simulink model "droop_model_with_current_limitation"  (R2018a)
settings: Solver=ode23tb  StartTime=0.0  StopTime=Tend  RelTol=1e-3
values from neighbouring files (symbols this model uses):
  C_4 = 0.1670*C_b    (= 1.00487241952e-06)    [VSM.m]    (also in dVOC.m; droop.m; droop_with_current_limitation.m; matching.m)
  C_6 = 0.2835*C_b    (= 1.70587623314e-06)    [VSM.m]    (also in dVOC.m; droop.m; droop_with_current_limitation.m; matching.m)
  C_8 = 0.2275*C_b    (= 1.36891302659e-06)    [VSM.m]    (also in dVOC.m; droop.m; droop_with_current_limitation.m; matching.m)
  C_dc = 0.008*(n)    (= 1.6)    [VSM.m]    (also in dVOC.m; droop.m; droop_with_current_limitation.m; matching.m)
  C_f = n*300*10^-6    (= 0.06)    [VSM.m]    (also in dVOC.m; droop.m; droop_with_current_limitation.m; matching.m)
  droop_percentage = 1    [VSM.m]    (also in dVOC.m; droop.m; droop_with_current_limitation.m; matching.m)
  I_b_LV = S_b/(sqrt(3)*V1_rms)    [VSM.m]    (also in dVOC.m; droop.m; droop_with_current_limitation.m = sqrt(2)*S_b/(sqrt(3)*V1_rms); matching.m)
  i_ll = -1.15*(S_b/Vdc_n)-i_loss_dc    [VSM.m]    (also in dVOC.m; droop.m; droop_with_current_limitation.m; matching.m)
  i_ul = 1.15*(S_b/Vdc_n)+i_loss_dc    [VSM.m]    (also in dVOC.m; droop.m; droop_with_current_limitation.m; matching.m)
  idppu = 0.9    [droop_with_current_limitation.m]
  isatpu = 1.2    [droop_with_current_limitation.m]
  k_dc = eta_1/(Vdc_n*m_p)    [VSM.m]    (also in dVOC.m; droop.m; droop_with_current_limitation.m; matching.m)
  K_dP = 2.3*S_b    (= 230000000)    [droop_with_current_limitation.m]
  K_p = (1/Vdc_n)    [VSM.m]    (also in dVOC.m; droop.m; droop_with_current_limitation.m; matching.m)
  K_r = 1/R_dc    [VSM.m]    (also in dVOC.m; droop.m; droop_with_current_limitation.m; matching.m)
  Kff_i = 1    [VSM.m]    (also in dVOC.m; droop.m; droop_with_current_limitation.m; matching.m)
  Kff_v = 1    [VSM.m]    (also in dVOC.m; droop.m; droop_with_current_limitation.m; matching.m)
  Ki_i = (1/n)*1.19    (= 0.00595)    [VSM.m]    (also in dVOC.m; droop.m; droop_with_current_limitation.m; matching.m)
  Ki_v = (n)*1.161022    (= 232.2044)    [VSM.m]    (also in dVOC.m; droop.m; droop_with_current_limitation.m; matching.m)
  ki_v_ac = 4*5.2500e-04    (= 0.0021)    [VSM.m]    (also in dVOC.m = 0.5; droop.m = 0.5; droop_with_current_limitation.m = 0.5; matching.m = 0.5)
  Kp_i = 0.738891    [VSM.m]    (also in dVOC.m; droop.m; droop_with_current_limitation.m; matching.m)
  Kp_v = 0.52    [VSM.m]    (also in dVOC.m; droop.m; droop_with_current_limitation.m; matching.m)
  kp_v_ac = 0.001    [VSM.m]    (also in dVOC.m; droop.m; droop_with_current_limitation.m; matching.m)
  L1_pu = 1*0.0186/m    (= 0.000186)    [VSM.m]    (also in dVOC.m; droop.m; droop_with_current_limitation.m; matching.m)
  L_45 = L_lines(2)    [VSM.m]    (also in dVOC.m; droop.m; droop_with_current_limitation.m; matching.m)
  L_56 = L_lines(3)    [VSM.m]    (also in dVOC.m; droop.m; droop_with_current_limitation.m; matching.m)
  L_67 = L_lines(5)    [VSM.m]    (also in dVOC.m; droop.m; droop_with_current_limitation.m; matching.m)
  L_78 = L_lines(6)    [VSM.m]    (also in dVOC.m; droop.m; droop_with_current_limitation.m; matching.m)
  L_89 = L_lines(8)    [VSM.m]    (also in dVOC.m; droop.m; droop_with_current_limitation.m; matching.m)
  L_94 = L_lines(9)    [VSM.m]    (also in dVOC.m; droop.m; droop_with_current_limitation.m; matching.m)
  L_f = (1/n)*200*10^-6    (= 1e-06)    [VSM.m]    (also in dVOC.m; droop.m; droop_with_current_limitation.m; matching.m)
  m_p = (2*pi*0.5)/(S_b)    (= 3.14159265359e-08)    [VSM.m]    (also in dVOC.m; droop.m; droop_with_current_limitation.m; matching.m)
  n = 200    [VSM.m]    (also in dVOC.m; droop.m; droop_with_current_limitation.m; matching.m)
  ps = base/3    (= 0.75)    [VSM.m]    (also in dVOC.m; droop.m; droop_with_current_limitation.m; matching.m)
  R1_pu = 1*0.00734/m    (= 7.34e-05)    [VSM.m]    (also in dVOC.m; droop.m; droop_with_current_limitation.m; matching.m)
  R_45 = R_lines(2)    [VSM.m]    (also in dVOC.m; droop.m; droop_with_current_limitation.m; matching.m)
  R_56 = R_lines(3)    [VSM.m]    (also in dVOC.m; droop.m; droop_with_current_limitation.m; matching.m)
  R_67 = R_lines(5)    [VSM.m]    (also in dVOC.m; droop.m; droop_with_current_limitation.m; matching.m)
  R_78 = R_lines(6)    [VSM.m]    (also in dVOC.m; droop.m; droop_with_current_limitation.m; matching.m)
  R_89 = R_lines(8)    [VSM.m]    (also in dVOC.m; droop.m; droop_with_current_limitation.m; matching.m)
  R_94 = R_lines(9)    [VSM.m]    (also in dVOC.m; droop.m; droop_with_current_limitation.m; matching.m)
  R_dc = (Vdc_n/(0.05*(S_b)/Vdc_n))    [VSM.m]    (also in dVOC.m; droop.m; droop_with_current_limitation.m; matching.m)
  R_f = 0.001/n    (= 5e-06)    [VSM.m]    (also in dVOC.m; droop.m; droop_with_current_limitation.m; matching.m)
  S_b = 100*(10^6)    (= 100000000)    [VSM.m]    (also in dVOC.m; droop.m; droop_with_current_limitation.m; matching.m)
  S_bt = S_b    (= 100000000)    [VSM.m]    (also in dVOC.m; droop.m; droop_with_current_limitation.m; matching.m)
  T_en = T_load-0.5    (= 24.5)    [VSM.m]    (also in dVOC.m; droop.m; droop_with_current_limitation.m; matching.m)
  T_load = 25    [VSM.m]    (also in dVOC.m; droop.m; droop_with_current_limitation.m; matching.m)
  T_loss = Tend    (= 50)    [dVOC.m]    (also in droop.m; droop_with_current_limitation.m)
  T_ms = 0.001    [dVOC.m]    (also in droop.m; droop_with_current_limitation.m)
  T_s = 1e-4    (= 0.0001)    [VSM.m]    (also in dVOC.m; droop.m; droop_with_current_limitation.m; matching.m)
  tau_dc = 0.05    [VSM.m]    (also in dVOC.m; droop.m; droop_with_current_limitation.m; matching.m)
  tau_g = 5    [VSM.m]    (also in dVOC.m; droop.m; droop_with_current_limitation.m; matching.m)
  V1_rms = 1000    [VSM.m]    (also in dVOC.m; droop.m; droop_with_current_limitation.m; matching.m)
  V2_rms = 13800    [VSM.m]    (also in dVOC.m; droop.m; droop_with_current_limitation.m; matching.m)
  V_m = sqrt(2/3)*V1_rms    [VSM.m]    (also in dVOC.m; droop.m; droop_with_current_limitation.m; matching.m)
  Vdc_n = 3*V_m    [VSM.m]    (also in dVOC.m; droop.m; droop_with_current_limitation.m; matching.m)
  w_b = 2*pi*f_b    (= 314.159265359)    [VSM.m]    (also in dVOC.m; droop.m; droop_with_current_limitation.m; matching.m)
  w_f = 2*pi*5    (= 31.4159265359)    [VSM.m]    (also in dVOC.m; droop.m; droop_with_current_limitation.m; matching.m)
undefined symbols (not defined in the file or in its folder): D1, Delta, i_dc
libraries: powerlib x88, powerlib_meascontrol x22, cstblocks x3, simulink x2, sps_avr x1
(part 1 of 2)
settings Model: SimulationMode=accelerator  ExtModeTrigDuration=100  Creator=TayyebiA  LastModifiedBy=TayyebiA
settings DataIOCC: SaveOutput=off  StateSaveName=tmp_raccel_xout  SignalLoggingName=tmp_raccel_logsout
settings OptimizationCC: EfficientMapNaN2IntZero=off
settings HardwareCC: TargetBitPerPointer=64  TargetBitPerSizeT=64  TargetBitPerPtrDiffT=64  TargetLongLongMode=on  TargetIntDivRoundTo=Zero  TargetEndianess=LittleEndian  TargetWordSize=64  TargetHWDeviceType=MATLAB Host  ProdEqTarget=off
settings CodeAppCC: MaxIdLength=128
settings GRTTargetCC: TargetLangStandard=C89/C90 (ANSI)  CombineOutputUpdateFcns=off  GRTInterface=on

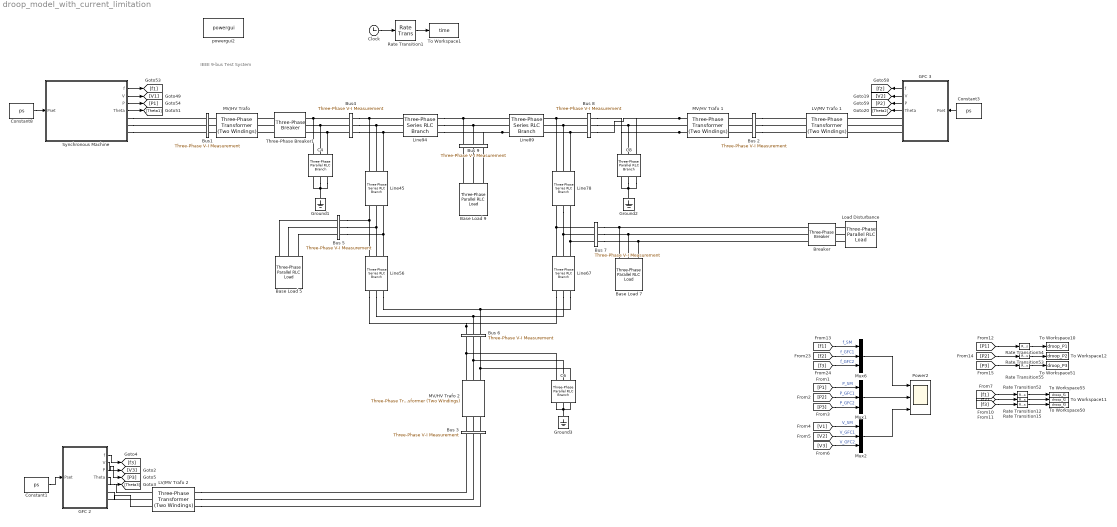
== system droop_model_with_current_limitation ==
  note: IEEE 9-bus Test System
  Base Load 5 : powerlib/Elements/Three-Phase Parallel RLC Load  LConnTagsString=A|B|C  Configuration=Y (grounded)  NominalVoltage=230e3  Vabc=[1e3 1e3 1e3]  Vabcp=[1e3 1e3 1e3]  NominalFrequency=50  UnbalancedPower=off  ActivePower=pl  InductivePower=0  CapacitivePower=0  Pabc=[10e3 9e3 11e3]  QLabc=[100 90 110]  QCabc=[100 90 110]  Pabcp=[10e3 9e3 11e3]  QLabcp=[100 90 110]  QCabcp=[100 90 110]  Measurements=None  LoadType=constant Z
  Base Load 7 : powerlib/Elements/Three-Phase Parallel RLC Load  LConnTagsString=A|B|C  Configuration=Y (grounded)  NominalVoltage=230e3  Vabc=[1e3 1e3 1e3]  Vabcp=[1e3 1e3 1e3]  NominalFrequency=50  UnbalancedPower=off  ActivePower=pl  InductivePower=0  CapacitivePower=0  Pabc=[10e3 9e3 11e3]  QLabc=[100 90 110]  QCabc=[100 90 110]  Pabcp=[10e3 9e3 11e3]  QLabcp=[100 90 110]  QCabcp=[100 90 110]  Measurements=None  LoadType=constant Z
  "Base Load 9 " : powerlib/Elements/Three-Phase Parallel RLC Load  LConnTagsString=A|B|C  Configuration=Y (grounded)  NominalVoltage=230e3  Vabc=[1e3 1e3 1e3]  Vabcp=[1e3 1e3 1e3]  NominalFrequency=50  UnbalancedPower=off  ActivePower=pl  InductivePower=0  CapacitivePower=0  Pabc=[10e3 9e3 11e3]  QLabc=[100 90 110]  QCabc=[100 90 110]  Pabcp=[10e3 9e3 11e3]  QLabcp=[100 90 110]  QCabcp=[100 90 110]  Measurements=None  LoadType=constant Z
  Breaker : powerlib/Elements/Three-Phase Breaker  InitialState=open  SwitchA=on  SwitchB=on  SwitchC=on  SwitchTimes=[T_load]  External=off  BreakerResistance=0.01  SnubberResistance=1e6  SnubberCapacitance=inf  Measurements=None
  Bus 2 : powerlib/Measurements/Three-Phase V-I Measurement  VoltageMeasurement=no  SetLabelV=on  LabelV=Vabc_8  Vpu=on  VpuLL=off  CurrentMeasurement=no  SetLabelI=on  LabelI=Iabc_8  Ipu=on  Pbase=S_b  Vbase=V_b  OutputType=Complex  PhasorSimulation=off  PSBequivalent=0
  Bus 3 : powerlib/Measurements/Three-Phase V-I Measurement  VoltageMeasurement=no  SetLabelV=off  LabelV=Vabc_6  Vpu=off  VpuLL=off  CurrentMeasurement=no  SetLabelI=off  LabelI=Iabc_6  Ipu=off  Pbase=S_b  Vbase=V_b  OutputType=Complex  PhasorSimulation=off  PSBequivalent=0
  Bus 5 : powerlib/Measurements/Three-Phase V-I Measurement  VoltageMeasurement=no  SetLabelV=on  LabelV=Vabc_5  Vpu=on  VpuLL=off  CurrentMeasurement=no  SetLabelI=on  LabelI=Iabc_5  Ipu=on  Pbase=S_b  Vbase=V_b  OutputType=Complex  PhasorSimulation=off  PSBequivalent=0
  Bus 6 : powerlib/Measurements/Three-Phase V-I Measurement  VoltageMeasurement=no  SetLabelV=off  LabelV=Vabc_6  Vpu=off  VpuLL=off  CurrentMeasurement=no  SetLabelI=off  LabelI=Iabc_6  Ipu=off  Pbase=S_b  Vbase=V_b  OutputType=Complex  PhasorSimulation=off  PSBequivalent=0
  Bus 7 : powerlib/Measurements/Three-Phase V-I Measurement  VoltageMeasurement=no  SetLabelV=on  LabelV=Vabc_5  Vpu=on  VpuLL=off  CurrentMeasurement=no  SetLabelI=on  LabelI=Iabc_5  Ipu=on  Pbase=S_b  Vbase=V_b  OutputType=Complex  PhasorSimulation=off  PSBequivalent=0
  Bus 8 : powerlib/Measurements/Three-Phase V-I Measurement  VoltageMeasurement=no  SetLabelV=on  LabelV=Vabc_8  Vpu=on  VpuLL=off  CurrentMeasurement=no  SetLabelI=on  LabelI=Iabc_8  Ipu=on  Pbase=S_b  Vbase=V_b  OutputType=Complex  PhasorSimulation=off  PSBequivalent=0
  Bus 9 : powerlib/Measurements/Three-Phase V-I Measurement  VoltageMeasurement=no  SetLabelV=on  LabelV=Vabc_9  Vpu=on  VpuLL=off  CurrentMeasurement=no  SetLabelI=on  LabelI=Iabc_9  Ipu=on  Pbase=S_b  Vbase=V_b  OutputType=Complex  PhasorSimulation=off  PSBequivalent=0
  Bus1 : powerlib/Measurements/Three-Phase V-I Measurement  VoltageMeasurement=no  SetLabelV=on  LabelV=Vabc_1  Vpu=on  VpuLL=off  CurrentMeasurement=no  SetLabelI=on  LabelI=Iabc_1  Ipu=on  Pbase=S_b  Vbase=V_b  OutputType=Complex  PhasorSimulation=off  PSBequivalent=0
  Bus4 : powerlib/Measurements/Three-Phase V-I Measurement  VoltageMeasurement=no  SetLabelV=on  LabelV=Vabc_4  Vpu=on  VpuLL=off  CurrentMeasurement=no  SetLabelI=on  LabelI=Iabc_4  Ipu=on  Pbase=S_b  Vbase=V_b  OutputType=Complex  PhasorSimulation=off  PSBequivalent=0
  C4 : powerlib/Elements/Three-Phase Parallel RLC Branch  LConnTagsString=A|B|C  RConnTagsString=A|B|C  BranchType=C  Resistance=1  Inductance=1e-3  Capacitance=C_4  Measurements=None
      settings: SourceProductName=Simscape Power Systems  SourceProductBaseCode=PS
  C6 : powerlib/Elements/Three-Phase Parallel RLC Branch  LConnTagsString=A|B|C  RConnTagsString=A|B|C  BranchType=C  Resistance=1  Inductance=1e-3  Capacitance=C_6  Measurements=None
      settings: SourceProductName=Simscape Power Systems  SourceProductBaseCode=PS
  C8 : powerlib/Elements/Three-Phase Parallel RLC Branch  LConnTagsString=A|B|C  RConnTagsString=A|B|C  BranchType=C  Resistance=1  Inductance=1e-3  Capacitance=C_8  Measurements=None
      settings: SourceProductName=Simscape Power Systems  SourceProductBaseCode=PS
  Clock : Clock
  Constant1 : Constant  Value=ps
  Constant3 : Constant  Value=ps
  Constant8 : Constant  Value=ps
  GFC 2 : Subsystem
  GFC 3 : Subsystem
  Ground1 : powerlib/Elements/Ground  LConnTagsString=a
  Ground2 : powerlib/Elements/Ground  LConnTagsString=a
  Ground3 : powerlib/Elements/Ground  LConnTagsString=a
  LV/MV Trafo 1 : powerlib/Elements/Three-Phase Transformer (Two Windings)  Winding1Connection=Yg  Winding2Connection=Yg  CoreType=Three single-phase transformers  SetSaturation=off  Hysteresis=off  DataFile='hysteresis'  SetInitialFlux=off  Measurements=None  UNITS=pu  NominalPower=[S_bt 50 ]  Winding1="[ V1_rms R1_pu  L1_pu]"  Winding2=[ V2_rms R1_pu L1_pu]  Rm=Rm_pu  Lm=Lm_pu  L0=0.5  Saturation="[ 0,0  ;  0.005,1.2  ;  1.0,1.4 ]"  InitialFluxes=[ 0.8 , -0.8 , 0.7 ]  MoreParameters=off  BreakLoop=off  DataType=off  TransfoNumber=0
  LV/MV Trafo 2 : powerlib/Elements/Three-Phase Transformer (Two Windings)  Winding1Connection=Yg  Winding2Connection=Yg  CoreType=Three single-phase transformers  SetSaturation=off  Hysteresis=off  DataFile='hysteresis'  SetInitialFlux=off  Measurements=None  UNITS=pu  NominalPower=[ S_bt 50 ]  Winding1="[ V1_rms R1_pu  L1_pu]"  Winding2=[ V2_rms R1_pu L1_pu]  Rm=Rm_pu  Lm=Lm_pu  L0=0.5  Saturation="[ 0,0  ;  0.005,1.2  ;  1.0,1.4 ]"  InitialFluxes=[ 0.8 , -0.8 , 0.7 ]  MoreParameters=off  BreakLoop=off  DataType=off  TransfoNumber=0
  Line45 : powerlib/Elements/Three-Phase Series RLC Branch  LConnTagsString=A|B|C  RConnTagsString=A|B|C  BranchType=RL  Resistance=R_45  Inductance=L_45  Capacitance=0  Measurements=None
  Line56 : powerlib/Elements/Three-Phase Series RLC Branch  LConnTagsString=A|B|C  RConnTagsString=A|B|C  BranchType=RL  Resistance=R_56  Inductance=L_56  Capacitance=0  Measurements=None
  Line67 : powerlib/Elements/Three-Phase Series RLC Branch  LConnTagsString=A|B|C  RConnTagsString=A|B|C  BranchType=RL  Resistance=R_67  Inductance=L_67  Capacitance=0  Measurements=None
  Line78 : powerlib/Elements/Three-Phase Series RLC Branch  LConnTagsString=A|B|C  RConnTagsString=A|B|C  BranchType=RL  Resistance=R_78  Inductance=L_78  Capacitance=0  Measurements=None
  Line89 : powerlib/Elements/Three-Phase Series RLC Branch  LConnTagsString=A|B|C  RConnTagsString=A|B|C  BranchType=RL  Resistance=R_89  Inductance=L_89  Capacitance=0  Measurements=None
  Line94 : powerlib/Elements/Three-Phase Series RLC Branch  LConnTagsString=A|B|C  RConnTagsString=A|B|C  BranchType=RL  Resistance=R_94  Inductance=L_94  Capacitance=0  Measurements=None
  Load Disturbance : powerlib/Elements/Three-Phase Parallel RLC Load  LConnTagsString=A|B|C  Configuration=Y (grounded)  NominalVoltage=230e3  Vabc=[1e3 1e3 1e3]  Vabcp=[1e3 1e3 1e3]  NominalFrequency=50  UnbalancedPower=off  ActivePower=load_step  InductivePower=0  CapacitivePower=0  Pabc=[10e3 9e3 11e3]  QLabc=[100 90 110]  QCabc=[100 90 110]  Pabcp=[10e3 9e3 11e3]  QLabcp=[100 90 110]  QCabcp=[100 90 110]  Measurements=None  LoadType=constant Z
  "MV/HV Trafo " : powerlib/Elements/Three-Phase Transformer (Two Windings)  Winding1Connection=Delta (D1)  Winding2Connection=Yg  CoreType=Three single-phase transformers  SetSaturation=off  Hysteresis=off  DataFile='hysteresis'  SetInitialFlux=off  Measurements=None  UNITS=pu  NominalPower=[ 210e6 50 ]  Winding1="[V2_rms 0.0027  0.08]"  Winding2=[230e3 0.0027 0.08]  Rm=500  Lm=500  L0=0.5  Saturation="[ 0,0  ;  0.005,1.2  ;  1.0,1.4 ]"  InitialFluxes=[ 0.8 , -0.8 , 0.7 ]  MoreParameters=off  BreakLoop=off  DataType=off  TransfoNumber=0
  "MV/HV Trafo 1 " : powerlib/Elements/Three-Phase Transformer (Two Windings)  Winding1Connection=Yg  Winding2Connection=Yg  CoreType=Three single-phase transformers  SetSaturation=off  Hysteresis=off  DataFile='hysteresis'  SetInitialFlux=off  Measurements=None  UNITS=pu  NominalPower=[ 210e6 50 ]  Winding1=[V2_rms 0.0027 0.08]  Winding2=[ 230e3 0.0027 0.08]  Rm=500  Lm=500  L0=0.5  Saturation="[ 0,0  ;  0.005,1.2  ;  1.0,1.4 ]"  InitialFluxes=[ 0.8 , -0.8 , 0.7 ]  MoreParameters=off  BreakLoop=off  DataType=off  TransfoNumber=0
  "MV/HV Trafo 2 " : powerlib/Elements/Three-Phase Transformer (Two Windings)  Winding1Connection=Yg  Winding2Connection=Yg  CoreType=Three single-phase transformers  SetSaturation=off  Hysteresis=off  DataFile='hysteresis'  SetInitialFlux=off  Measurements=None  UNITS=pu  NominalPower=[ 210e6 50 ]  Winding1=[V2_rms 0.0027 0.08]  Winding2=[230e3 0.0027 0.08]  Rm=500  Lm=500  L0=0.5  Saturation="[ 0,0  ;  0.005,1.2  ;  1.0,1.4 ]"  InitialFluxes=[ 0.8 , -0.8 , 0.7 ]  MoreParameters=off  BreakLoop=off  DataType=off  TransfoNumber=0
  Mux1 : Mux  Inputs=3
  Mux2 : Mux  Inputs=3
  Mux6 : Mux  Inputs=3
  Power2 : Scope  NumInputPorts=3
  Rate Transition1 : RateTransition  OutPortSampleTime=0.001
  Rate Transition{12,15,52..55} (6 alike) : RateTransition  OutPortSampleTime=T_ms
  Synchronous Machine : Subsystem
  Three-Phase Breaker1 : powerlib/Elements/Three-Phase Breaker  InitialState=closed  SwitchA=on  SwitchB=on  SwitchC=on  SwitchTimes=[T_loss]  External=off  BreakerResistance=1  SnubberResistance=1e6  SnubberCapacitance=inf  Measurements=None
  To Workspace1 : ToWorkspace  VariableName=time  SampleTime=T_ms
  To Workspace10 : ToWorkspace  VariableName=droop_P1  SampleTime=-1
  To Workspace11 : ToWorkspace  VariableName=droop_f2  SampleTime=-1
  To Workspace12 : ToWorkspace  VariableName=droop_P2  SampleTime=-1
  To Workspace50 : ToWorkspace  VariableName=droop_f3  SampleTime=-1
  To Workspace51 : ToWorkspace  VariableName=droop_P3  SampleTime=-1
  To Workspace55 : ToWorkspace  VariableName=droop_f1  SampleTime=-1
  powergui2 : powerlib/powergui  Priority=1  SimulationMode=Discrete  SampleTime=T_s  frequency=50  Iterations=50  frequencyindice=0  Pbase=100e6  ErrMax=0.0001  UnitsV=kV  UnitsW=MW  buscounter=0  FunctionMessages=off  echomessages=off  EnableUseOfTLC=off  CurrentSourceSwitches=off  DisableSnubberDevices=off  DisableRonSwitches=off  DisableVfSwitches=off  DisplayEquations=off  SolverType=Tustin/Backward Euler (TBE)  Interpol=off  ExternalGateDelay=off  methode=off  Ts=100  x0status=blocks  SPID=off  SwTol=0  HookPort=off  RestoreLinks=warning  ResistiveCurrentMeasurement=off  Frange=[0:2:500]  Ylog=off  Xlog=on  ShowGrid=off  save=off  variable=ZData  structure=0  ZoomFFT=off  StartTime=0.0  cycles=1  DisplayStyle=1  fundamental=60  FreqAxis=off  MaxFrequency=1000  frequencyindicesteady=1  RmsSteady=1  display=off
  wires:
  Constant3/1 -> GFC 3/1(Pset)
  Constant8/1 -> Synchronous Machine/1(Pset)
  Synchronous Machine/1(f) -> [f1]
  Synchronous Machine/2(V) -> [V1]
  Synchronous Machine/3(P) -> [P1]
  Synchronous Machine/4(Theta) -> [Theta1]
  [f1] -> Mux6/1  "f_SM"
  [f2] -> Mux6/2  "f_GFC1"
  [f3] -> Mux6/3  "f_GFC2"
  [P1] -> Mux1/1  "P_SM"
  [P3] -> Mux1/3  "P_GFC2"
  [P2] -> Mux1/2  "P_GFC1"
  [V2] -> Mux2/2  "V_GFC1"
  [V1] -> Mux2/1  "V_SM"
  [V3] -> Mux2/3  "V_GFC2"
  Mux6/1 -> Power2/1
  Mux1/1 -> Power2/2
  Mux2/1 -> Power2/3
  GFC 3/1(f) -> [f2]
  GFC 3/2(V) -> [V2]
  GFC 3/3(P) -> [P2]
  GFC 3/4(Theta) -> [Theta2]
  GFC 2/1(f) -> [f3]
  GFC 2/2(V) -> [V3]
  GFC 2/3(P) -> [P3]
  Constant1/1 -> GFC 2/1(Pset)
  GFC 2/4(Theta) -> [Theta3]
  [P3] -> Rate Transition55/1
  Rate Transition54/1 -> To Workspace10/1
  Rate Transition55/1 -> To Workspace51/1
  Rate Transition52/1 -> To Workspace55/1
  Rate Transition15/1 -> To Workspace50/1
  Rate Transition12/1 -> To Workspace11/1
  [f2] -> Rate Transition12/1
  [f3] -> Rate Transition15/1
  Rate Transition53/1 -> To Workspace12/1
  [P1] -> Rate Transition54/1
  [f1] -> Rate Transition52/1
  [P2] -> Rate Transition53/1
  Clock/1 -> Rate Transition1/1
  Rate Transition1/1 -> To Workspace1/1
  connections:
  "MV/HV Trafo 2 "/RConn2 -- Bus 6/RConn2 -- C6/LConn2
  Breaker/LConn2 -- Base Load 7/LConn2 -- Bus 7/LConn2
  Bus 8/RConn2 -- Line78/LConn2 -- Line89/RConn2
  GFC 3/RConn3 -- LV/MV Trafo 1/LConn1
  "MV/HV Trafo 1 "/RConn3 -- C8/LConn3 -- Bus 8/LConn3
  Line94/RConn2 -- Line89/LConn2 -- Bus 9/RConn2
  Bus 6/LConn1 -- Line56/RConn1 -- Line67/RConn1
  Breaker/LConn3 -- Base Load 7/LConn3 -- Bus 7/LConn3
  Line67/LConn1 -- Bus 7/RConn1 -- Line78/RConn1
  Line56/LConn3 -- Bus 5/LConn3 -- Line45/RConn3
  Bus 9/RConn3 -- Line89/LConn1 -- Line94/RConn1
  C4/RConn2 -- C4/RConn1 -- C4/RConn3 -- Ground1/LConn1
  "MV/HV Trafo 1 "/RConn1 -- C8/LConn1 -- Bus 8/LConn1
  Bus 8/LConn2 -- C8/LConn2 -- "MV/HV Trafo 1 "/RConn2
  C8/RConn3 -- Ground2/LConn1 -- C8/RConn1 -- C8/RConn2
  Line67/RConn2 -- Line56/RConn2 -- Bus 6/LConn2
  C4/LConn1 -- Three-Phase Breaker1/RConn1 -- Bus4/RConn1
  Bus4/LConn1 -- Line45/LConn1 -- Line94/LConn1
  C6/LConn3 -- Bus 6/RConn3 -- "MV/HV Trafo 2 "/RConn3
  GFC 3/RConn1 -- LV/MV Trafo 1/LConn3
  "MV/HV Trafo 2 "/RConn1 -- Bus 6/RConn1 -- C6/LConn1
  Bus4/LConn2 -- Line45/LConn2 -- Line94/LConn2
  Bus 8/RConn3 -- Line78/LConn3 -- Line89/RConn3
  Bus 8/RConn1 -- Line78/LConn1 -- Line89/RConn1
  Bus4/RConn3 -- Three-Phase Breaker1/RConn3 -- C4/LConn3
  Line56/LConn1 -- Bus 5/LConn1 -- Line45/RConn1
  Line89/LConn3 -- Bus 9/RConn1 -- Line94/RConn3
  Line67/RConn3 -- Line56/RConn3 -- Bus 6/LConn3
  GFC 3/RConn2 -- LV/MV Trafo 1/LConn2
  Bus4/LConn3 -- Line45/LConn3 -- Line94/LConn3
  Bus4/RConn2 -- Three-Phase Breaker1/RConn2 -- C4/LConn2
  Line56/LConn2 -- Bus 5/LConn2 -- Line45/RConn2
  "Base Load 9 "/LConn1 -- Bus 9/LConn3
  Base Load 5/LConn3 -- Bus 5/RConn3
  "Base Load 9 "/LConn3 -- Bus 9/LConn1
  Base Load 5/LConn1 -- Bus 5/RConn1
  Base Load 5/LConn2 -- Bus 5/RConn2
  "Base Load 9 "/LConn2 -- Bus 9/LConn2
  Load Disturbance/LConn3 -- Breaker/RConn3
  Load Disturbance/LConn2 -- Breaker/RConn2
  Load Disturbance/LConn1 -- Breaker/RConn1
  Bus1/LConn1 -- "MV/HV Trafo "/LConn1
  Bus1/LConn2 -- "MV/HV Trafo "/LConn2
  Bus1/LConn3 -- "MV/HV Trafo "/LConn3
  Synchronous Machine/RConn1 -- Bus1/RConn1
  Synchronous Machine/RConn2 -- Bus1/RConn2
  Synchronous Machine/RConn3 -- Bus1/RConn3
  LV/MV Trafo 2/RConn1 -- Bus 3/RConn1
  LV/MV Trafo 2/RConn2 -- Bus 3/RConn2
  LV/MV Trafo 2/RConn3 -- Bus 3/RConn3
  Bus 3/LConn1 -- "MV/HV Trafo 2 "/LConn1
  Bus 3/LConn2 -- "MV/HV Trafo 2 "/LConn2
  Bus 3/LConn3 -- "MV/HV Trafo 2 "/LConn3
  Bus 2/LConn1 -- LV/MV Trafo 1/RConn3
  Bus 2/LConn2 -- LV/MV Trafo 1/RConn2
  Bus 2/LConn3 -- LV/MV Trafo 1/RConn1
  Bus 2/RConn3 -- "MV/HV Trafo 1 "/LConn1
  Bus 2/RConn2 -- "MV/HV Trafo 1 "/LConn2
  Bus 2/RConn1 -- "MV/HV Trafo 1 "/LConn3
  Breaker/LConn1 -- Bus 7/LConn1 -- Base Load 7/LConn1
  Line67/LConn3 -- Bus 7/RConn3 -- Line78/RConn3
  Line78/RConn2 -- Bus 7/RConn2 -- Line67/LConn2
  C6/RConn1 -- C6/RConn3 -- Ground3/LConn1 -- C6/RConn2
  GFC 2/RConn1 -- LV/MV Trafo 2/LConn1
  GFC 2/RConn2 -- LV/MV Trafo 2/LConn2
  GFC 2/RConn3 -- LV/MV Trafo 2/LConn3
  Three-Phase Breaker1/LConn1 -- "MV/HV Trafo "/RConn1
  Three-Phase Breaker1/LConn2 -- "MV/HV Trafo "/RConn2
  Three-Phase Breaker1/LConn3 -- "MV/HV Trafo "/RConn3

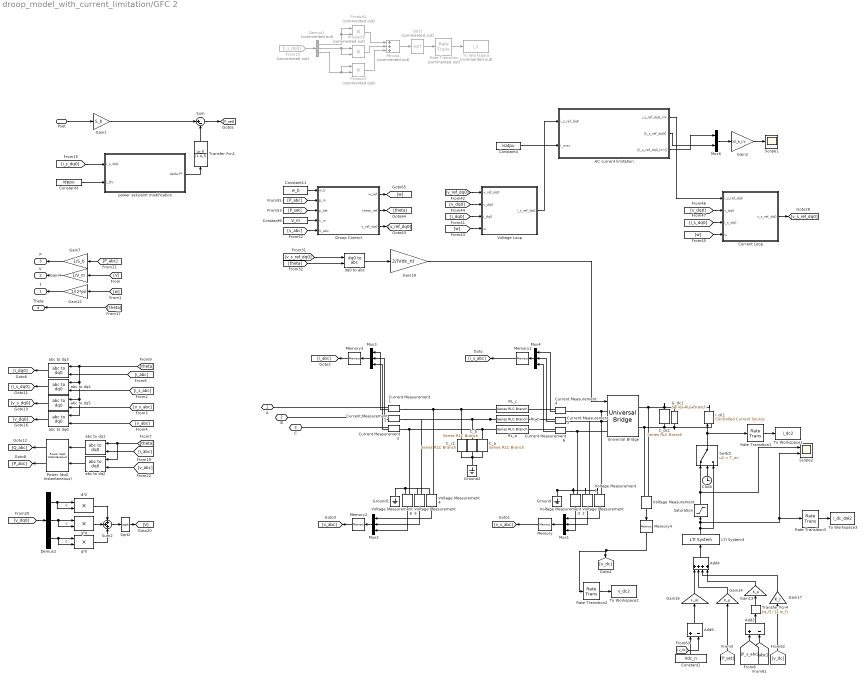
== system droop_model_with_current_limitation/GFC 2 ==
  Pset : Inport
  AC current limitation : Subsystem
  Add2 : Sum  Inputs=+-
  Add4 : Sum  Inputs=++++
  Add6 : Sum  Inputs=+-
  C_a : powerlib/Elements/Series RLC Branch  LConnTagsString=__new0  RConnTagsString=__new0  BranchType=C  Resistance=1  Inductance=1e-3  SetiL0=off  InitialCurrent=0  Capacitance=C_f  Setx0=off  InitialVoltage=165  Measurements=None
  C_b : powerlib/Elements/Series RLC Branch  LConnTagsString=__new0  RConnTagsString=__new0  BranchType=C  Resistance=1  Inductance=1e-3  SetiL0=off  InitialCurrent=0  Capacitance=C_f  Setx0=off  InitialVoltage=165  Measurements=None
  C_c1 : powerlib/Elements/Series RLC Branch  LConnTagsString=__new0  RConnTagsString=__new0  BranchType=C  Resistance=1  Inductance=1e-3  SetiL0=off  InitialCurrent=0  Capacitance=C_f  Setx0=off  InitialVoltage=165  Measurements=None
  C_dc1 : powerlib/Elements/Series RLC Branch  LConnTagsString=__new0  RConnTagsString=__new0  BranchType=C  Resistance=0.01  Inductance=1e-3  SetiL0=off  InitialCurrent=0  Capacitance=C_dc  Setx0=off  InitialVoltage=Vdc_n  Measurements=None
  Clock : Clock
  Constant1 : Constant  Value=Vdc_n
  Constant11 : Constant  Value=w_b
  Constant3 : Constant  Value=idppu
  Constant4 : Constant  Value=isatpu
  Constant9 : Constant  Value=V_m
  Current Loop : Subsystem
  Current Measurement{1..6} (6 alike) : powerlib/Measurements/Current Measurement  PhasorSimulation=off  OutputType=Complex  PSBequivalent=0
  Demux1 : Demux  Commented=on  Outputs=3
  Demux2 : Demux  Outputs=3
  Droop Control : Subsystem
  From10 : From  Commented=on  GotoTag=i_s_dq0
  G_dc1 : powerlib/Elements/Series RLC Branch  LConnTagsString=__new0  RConnTagsString=__new0  BranchType=R  Resistance=R_dc  Inductance=1e-3  SetiL0=off  InitialCurrent=0  Capacitance=1e-6  Setx0=off  InitialVoltage=0  Measurements=None
  Gain1 : Gain  Gain=S_b
  Gain12 : Gain  Gain=1/(2*pi)
  Gain13 : Gain  Gain=K_p
  Gain14 : Gain  Gain=K_p
  Gain16 : Gain  Gain=k_dc
  Gain17 : Gain  Gain=K_r
  Gain19 : Gain  Gain=2/(Vdc_n)
  Gain2 : Gain  Gain=1/I_b_LV
  Gain4 : Gain  Gain=1/V_m
  Gain7 : Gain  Gain=1/S_b
  Ground : powerlib/Elements/Ground  LConnTagsString=a
  Ground1 : powerlib/Elements/Ground  LConnTagsString=a
  Ground2 : powerlib/Elements/Ground  LConnTagsString=a
  LTI System3 : cstblocks/LTI System  sys=tf(1,[tau_dc 1])  IC=[]
  Memory{,1..4} (5 alike) : Memory
  Minus4 : Sum  Commented=on  Inputs=+++
  Mux{1..4} (4 alike) : Mux  Inputs=3
  Mux6 : Mux  Inputs=2
  "Power (dq0, Instantaneous)" : powerlib_meascontrol/Measurements/Power (dq0, Instantaneous)
      settings: SourceProductName=Simscape Power Systems  SourceProductBaseCode=PS
  Product1 : Product  Commented=on  RndMeth=Zero
  Product2 : Product  Commented=on  RndMeth=Zero
  Product7 : Product  Commented=on  RndMeth=Zero
  RL_a : powerlib/Elements/Series RLC Branch  LConnTagsString=__new0  RConnTagsString=__new0  BranchType=RL  Resistance=R_f  Inductance=L_f  SetiL0=off  InitialCurrent=0  Capacitance=1e-6  Setx0=off  InitialVoltage=0  Measurements=Branch voltage and current
  RL_b : powerlib/Elements/Series RLC Branch  LConnTagsString=__new0  RConnTagsString=__new0  BranchType=RL  Resistance=R_f  Inductance=L_f  SetiL0=off  InitialCurrent=0  Capacitance=1e-6  Setx0=off  InitialVoltage=0  Measurements=None
  RL_c : powerlib/Elements/Series RLC Branch  LConnTagsString=__new0  RConnTagsString=__new0  BranchType=RL  Resistance=R_f  Inductance=L_f  SetiL0=off  InitialCurrent=0  Capacitance=1e-6  Setx0=off  InitialVoltage=0  Measurements=None
  Rate Transition : RateTransition  Commented=on  OutPortSampleTime=0.001
  Rate Transition1 : RateTransition  OutPortSampleTime=0.001
  Rate Transition2 : RateTransition  OutPortSampleTime=0.001
  Rate Transition3 : RateTransition  OutPortSampleTime=0.001
  Saturation : Saturate  UpperLimit=i_ul  LowerLimit=i_ll
  Scope1 : Scope
  Scope2 : Scope  NumInputPorts=2
  Sqrt1 : Sqrt  Commented=on  SaturateOnIntegerOverflow=on
  Sqrt2 : Sqrt  SaturateOnIntegerOverflow=on
  Sum : Sum  Inputs=|+-
  Sum2 : Sum  Inputs=+++  SaturateOnIntegerOverflow=on  InputSameDT=on  OutDataTypeStr=Inherit: Same as first input
  Switch : Switch  Criteria=u2 > Threshold  Threshold=T_en
  To Workspace : ToWorkspace  Commented=on  VariableName=i_2  SampleTime=-1
  To Workspace1 : ToWorkspace  VariableName=i_dc2  SampleTime=-1
  To Workspace2 : ToWorkspace  VariableName=v_dc2  SampleTime=-1
  To Workspace3 : ToWorkspace  VariableName=i_dc_del2  SampleTime=-1
  Transfer Fcn1 : TransferFcn  Numerator=[w_f]  Denominator=[1 w_f]
  Transfer Fcn4 : TransferFcn  Numerator=[w_f]  Denominator=[1 w_f]
  Universal Bridge : powerlib/Power Electronics/Universal Bridge  Arms=3  SnubberResistance=1e5  SnubberCapacitance=inf  Device=Average-model based VSC  Ron=1e-3  Lon=0  ForwardVoltages="[  0  0  ]"  ForwardVoltage=0  GTOparameters=[ 10e-6 , 20e-6 ]  IGBTparameters=[ 1e-6 , 2e-6 ]  Measurements=None  Measurements_2=None  converterType=Rectifier
  Voltage Loop : Subsystem
  Voltage Measurement{,1..6} (7 alike) : powerlib/Measurements/Voltage Measurement  PhasorSimulation=off  OutputType=Complex  PSBequivalent=0
  abc to dq{1..6} (6 alike) : powerlib_meascontrol/Transformations/abc to dq0  Alignment=90 degrees behind phase A axis
  dq0 to abc : powerlib_meascontrol/Transformations/dq0 to abc  Alignment=90 degrees behind phase A axis
  d²2 : Product  SaturateOnIntegerOverflow=on  RndMeth=Zero  InputSameDT=on  OutDataTypeStr=Inherit: Same as first input
  i_dc1 : powerlib/Electrical Sources/Controlled Current Source  Initialize=off  Source_Type=DC  Amplitude=i_dc  Phase=0  Frequency=0  Measurements=None
  power set-point modification : Subsystem
  q²4 : Product  SaturateOnIntegerOverflow=on  RndMeth=Zero  InputSameDT=on  OutDataTypeStr=Inherit: Same as first input
  q²5 : Product  SaturateOnIntegerOverflow=on  RndMeth=Zero  InputSameDT=on  OutDataTypeStr=Inherit: Same as first input
  A : PMIOPort  Side=Right
  B : PMIOPort  Port=2  Side=Right
  C : PMIOPort  Port=3  Side=Right
  f : Outport
  V : Outport  Port=2
  P : Outport  Port=3
  Theta : Outport  Port=4
  wires:
  Product2/1 -> Minus4/2
  Sqrt1/1 -> Rate Transition/1
  Rate Transition/1 -> To Workspace/1
  Product7/1 -> Minus4/3
  Demux1/2 -> Product2/2, Product2/1
  Minus4/1 -> Sqrt1/1
  Demux1/3 -> Product7/2, Product7/1
  Product1/1 -> Minus4/1
  Demux1/1 -> Product1/1, Product1/2
  From10/1 -> Demux1/1
  Add4/1 -> LTI System3/1
  Clock/1 -> Switch/2
  Saturation/1 -> Scope2/1, Switch/1
  LTI System3/1 -> Switch/3, Rate Transition3/1, Scope2/2, Saturation/1
  Gain7/1 -> P/1
  [P_abc] -> Gain7/1
  Current Measurement6/1 -> Mux4/3
  Current Measurement5/1 -> Mux4/2
  Current Measurement4/1 -> Mux4/1
  Current Measurement3/1 -> Mux3/3
  Current Measurement2/1 -> Mux3/2
  Current Measurement1/1 -> Mux3/1
  Voltage Measurement4/1 -> Mux2/1
  Voltage Measurement5/1 -> Mux2/2
  Voltage Measurement6/1 -> Mux2/3
  Voltage Measurement3/1 -> Mux1/3
  Voltage Measurement2/1 -> Mux1/2
  Voltage Measurement1/1 -> Mux1/1
  [V] -> Gain4/1
  Gain12/1 -> f/1
  [w] -> Gain12/1
  Mux2/1 -> Memory2/1
  Mux3/1 -> Memory3/1
  Mux1/1 -> Memory/1
  abc to dq1/1 -> "Power (dq0, Instantaneous)"/2
  abc to dq2/1 -> "Power (dq0, Instantaneous)"/1
  [theta] -> abc to dq2/2, abc to dq1/2
  [v_abc] -> abc to dq2/1
  "Power (dq0, Instantaneous)"/2 -> [Q_abc]
  "Power (dq0, Instantaneous)"/1 -> [P_abc]
  [i_abc] -> abc to dq1/1
  Gain4/1 -> V/1
  [theta] -> Theta/1
  [i_abc] -> abc to dq3/1
  [i_s_abc] -> abc to dq4/1
  [v_abc] -> abc to dq6/1
  [v_s_abc] -> abc to dq5/1
  [theta] -> abc to dq4/2, abc to dq5/2, abc to dq6/2, abc to dq3/2
  abc to dq3/1 -> [i_dq0]
  abc to dq4/1 -> [i_s_dq0]
  abc to dq5/1 -> [v_s_dq0]
  abc to dq6/1 -> [v_dq0]
  [theta] -> dq0 to abc/2
  q²4/1 -> Sum2/2
  [v_dq0] -> Demux2/1
  q²5/1 -> Sum2/3
  Sum2/1 -> Sqrt2/1
  Demux2/3 -> q²5/1, q²5/2  "0"
  d²2/1 -> Sum2/1
  Demux2/2 -> q²4/1, q²4/2  "q"
  Demux2/1 -> d²2/1, d²2/2  "d"
  Sqrt2/1 -> [V]
  Mux4/1 -> Memory1/1
  Memory2/1 -> [v_abc]
  Memory3/1 -> [i_abc]
  Voltage Measurement/1 -> Memory4/1
  Memory4/1 -> Rate Transition2/1, [v_dc]
  Memory/1 -> [v_s_abc]
  Memory1/1 -> [i_s_abc]
  dq0 to abc/1 -> Gain19/1
  [w] -> Current Loop/4(w)
  [v_ref_dq0] -> Voltage Loop/1(v_ref_dq0)
  [i_dq0] -> Voltage Loop/3(i_dq0)
  [v_dq0] -> Current Loop/2(v_dq0)
  [i_s_dq0] -> Current Loop/3(i_s_dq0)
  Current Loop/1(v_s_ref_dq0) -> [v_s_ref_dq0]
  [w] -> Voltage Loop/4(w)
  [v_dq0] -> Voltage Loop/2(v_dq0)
  Gain19/1 -> Universal Bridge/1
  [v_s_ref_dq0] -> dq0 to abc/1
  Constant11/1 -> Droop Control/1(w_b)
  Droop Control/3(v_ref_dq0) -> [v_ref_dq0]
  [P_abc] -> Droop Control/2(p_m)
  Constant9/1 -> Droop Control/4(v_m)
  [v_abc] -> Droop Control/5(V_abc)
  Droop Control/2(theta_ref) -> [theta]
  Droop Control/1(w_ref) -> [w]
  [P_set] -> Droop Control/3(p_set)
  [P_abc] -> Add2/2
  Gain14/1 -> Add4/4
  [P_set] -> Gain13/1
  Gain13/1 -> Add4/2
  Gain16/1 -> Add4/1
  Constant1/1 -> Add6/1
  Gain17/1 -> Add4/3
  [v_dc] -> Add6/2
  Add6/1 -> Gain16/1
  [P_s_abc] -> Add2/1
  [v_dc] -> Gain17/1
  Pset/1 -> Gain1/1
  Gain1/1 -> Sum/1
  power set-point modification/1(delta P*) -> Transfer Fcn1/1
  [i_s_dq0] -> power set-point modification/1(i_s_dq0)
  Transfer Fcn4/1 -> Gain14/1
  Add2/1 -> Transfer Fcn4/1
  Mux6/1 -> Gain2/1
  Gain2/1 -> Scope1/1
  AC current limitation/1(i_s_ref_dq0_lim) -> Current Loop/1(i_s_ref_dq0)
  Voltage Loop/1(i_s_ref_dq0) -> AC current limitation/1(i_s_ref_dq0)
  AC current limitation/2(||i_s_ref_dq0||) -> Mux6/2
  Constant4/1 -> AC current limitation/2(i_max)
  AC current limitation/3(||i_s_ref_dq0_lim||) -> Mux6/1
  Sum/1 -> [P_set]
  Constant3/1 -> power set-point modification/2(i_thr)
  Transfer Fcn1/1 -> Sum/2
  Rate Transition1/1 -> To Workspace1/1
  Switch/1 -> Rate Transition1/1, i_dc1/1
  Rate Transition2/1 -> To Workspace2/1
  Rate Transition3/1 -> To Workspace3/1
  connections:
  RL_b/RConn1 -- Voltage Measurement5/LConn1 -- Current Measurement2/LConn1 -- C_b/LConn1
  Voltage Measurement6/LConn1 -- Current Measurement3/LConn1 -- C_a/LConn1 -- RL_a/RConn1
  Current Measurement4/RConn1 -- RL_c/LConn1
  Current Measurement6/RConn1 -- RL_a/LConn1
  Current Measurement5/RConn1 -- RL_b/LConn1
  Voltage Measurement/LConn1 -- Universal Bridge/RConn1 -- C_dc1/LConn1 -- G_dc1/LConn1 -- i_dc1/RConn1
  Voltage Measurement6/LConn2 -- Voltage Measurement5/LConn2 -- Voltage Measurement4/LConn2 -- Ground1/LConn1
  Ground/LConn1 -- Voltage Measurement2/LConn2 -- Voltage Measurement1/LConn2 -- Voltage Measurement3/LConn2
  Current Measurement3/RConn1 -- C/RConn1
  Current Measurement2/RConn1 -- B/RConn1
  Current Measurement1/RConn1 -- A/RConn1
  Current Measurement6/LConn1 -- Universal Bridge/LConn3 -- Voltage Measurement3/LConn1
  Universal Bridge/LConn2 -- Current Measurement5/LConn1 -- Voltage Measurement2/LConn1
  Universal Bridge/LConn1 -- Current Measurement4/LConn1 -- Voltage Measurement1/LConn1
  Universal Bridge/RConn2 -- Voltage Measurement/LConn2 -- C_dc1/RConn1 -- G_dc1/RConn1 -- i_dc1/LConn1
  C_b/RConn1 -- C_a/RConn1 -- Ground2/LConn1 -- C_c1/RConn1
  Voltage Measurement4/LConn1 -- Current Measurement1/LConn1 -- C_c1/LConn1 -- RL_c/RConn1

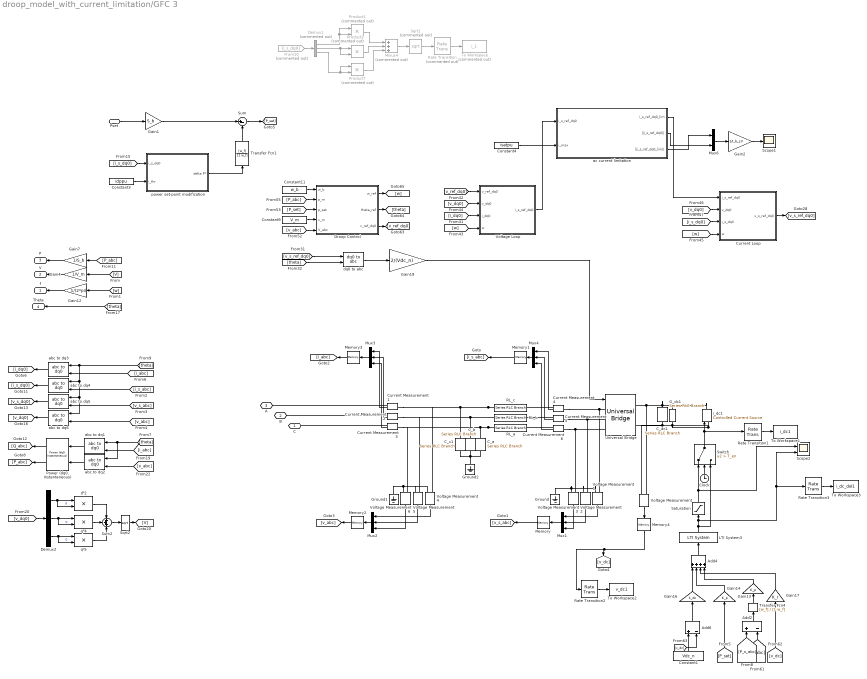
== system droop_model_with_current_limitation/GFC 3 ==
  Pset : Inport
  Add2 : Sum  Inputs=+-
  Add4 : Sum  Inputs=++++
  Add6 : Sum  Inputs=+-
  C_a : powerlib/Elements/Series RLC Branch  LConnTagsString=__new0  RConnTagsString=__new0  BranchType=C  Resistance=1  Inductance=1e-3  SetiL0=off  InitialCurrent=0  Capacitance=C_f  Setx0=off  InitialVoltage=165  Measurements=None
  C_b : powerlib/Elements/Series RLC Branch  LConnTagsString=__new0  RConnTagsString=__new0  BranchType=C  Resistance=1  Inductance=1e-3  SetiL0=off  InitialCurrent=0  Capacitance=C_f  Setx0=off  InitialVoltage=165  Measurements=None
  C_c1 : powerlib/Elements/Series RLC Branch  LConnTagsString=__new0  RConnTagsString=__new0  BranchType=C  Resistance=1  Inductance=1e-3  SetiL0=off  InitialCurrent=0  Capacitance=C_f  Setx0=off  InitialVoltage=165  Measurements=None
  C_dc1 : powerlib/Elements/Series RLC Branch  LConnTagsString=__new0  RConnTagsString=__new0  BranchType=C  Resistance=0.01  Inductance=1e-3  SetiL0=off  InitialCurrent=0  Capacitance=C_dc  Setx0=off  InitialVoltage=Vdc_n  Measurements=None
  Clock : Clock
  Constant1 : Constant  Value=Vdc_n
  Constant11 : Constant  Value=w_b
  Constant3 : Constant  Value=idppu
  Constant4 : Constant  Value=isatpu
  Constant9 : Constant  Value=V_m
  Current Loop : Subsystem
  Current Measurement{1..6} (6 alike) : powerlib/Measurements/Current Measurement  PhasorSimulation=off  OutputType=Complex  PSBequivalent=0
  Demux1 : Demux  Commented=on  Outputs=3
  Demux2 : Demux  Outputs=3
  Droop Control : Subsystem
  From10 : From  Commented=on  GotoTag=i_s_dq0
  G_dc1 : powerlib/Elements/Series RLC Branch  LConnTagsString=__new0  RConnTagsString=__new0  BranchType=R  Resistance=R_dc  Inductance=1e-3  SetiL0=off  InitialCurrent=0  Capacitance=1e-6  Setx0=off  InitialVoltage=0  Measurements=None
  Gain1 : Gain  Gain=S_b
  Gain12 : Gain  Gain=1/(2*pi)
  Gain13 : Gain  Gain=K_p
  Gain14 : Gain  Gain=K_p
  Gain16 : Gain  Gain=k_dc
  Gain17 : Gain  Gain=K_r
  Gain19 : Gain  Gain=2/(Vdc_n)
  Gain2 : Gain  Gain=1/I_b_LV
  Gain4 : Gain  Gain=1/V_m
  Gain7 : Gain  Gain=1/S_b
  Ground : powerlib/Elements/Ground  LConnTagsString=a
  Ground1 : powerlib/Elements/Ground  LConnTagsString=a
  Ground2 : powerlib/Elements/Ground  LConnTagsString=a
  LTI System3 : cstblocks/LTI System  sys=tf(1,[tau_dc 1])  IC=[]
  Memory{,1..4} (5 alike) : Memory
  Minus4 : Sum  Commented=on  Inputs=+++
  Mux{1..4} (4 alike) : Mux  Inputs=3
  Mux6 : Mux  Inputs=2
  "Power (dq0, Instantaneous)" : powerlib_meascontrol/Measurements/Power (dq0, Instantaneous)
      settings: SourceProductName=Simscape Power Systems  SourceProductBaseCode=PS
  Product1 : Product  Commented=on  RndMeth=Zero
  Product2 : Product  Commented=on  RndMeth=Zero
  Product7 : Product  Commented=on  RndMeth=Zero
  RL_a : powerlib/Elements/Series RLC Branch  LConnTagsString=__new0  RConnTagsString=__new0  BranchType=RL  Resistance=R_f  Inductance=L_f  SetiL0=off  InitialCurrent=0  Capacitance=1e-6  Setx0=off  InitialVoltage=0  Measurements=Branch voltage and current
  RL_b : powerlib/Elements/Series RLC Branch  LConnTagsString=__new0  RConnTagsString=__new0  BranchType=RL  Resistance=R_f  Inductance=L_f  SetiL0=off  InitialCurrent=0  Capacitance=1e-6  Setx0=off  InitialVoltage=0  Measurements=None
  RL_c : powerlib/Elements/Series RLC Branch  LConnTagsString=__new0  RConnTagsString=__new0  BranchType=RL  Resistance=R_f  Inductance=L_f  SetiL0=off  InitialCurrent=0  Capacitance=1e-6  Setx0=off  InitialVoltage=0  Measurements=None
  Rate Transition : RateTransition  Commented=on  OutPortSampleTime=0.001
  Rate Transition1 : RateTransition  OutPortSampleTime=0.001
  Rate Transition2 : RateTransition  OutPortSampleTime=0.001
  Rate Transition3 : RateTransition  OutPortSampleTime=0.001
  Saturation : Saturate  UpperLimit=i_ul  LowerLimit=i_ll
  Scope1 : Scope
  Scope2 : Scope  NumInputPorts=2
  Sqrt1 : Sqrt  Commented=on  SaturateOnIntegerOverflow=on
  Sqrt2 : Sqrt  SaturateOnIntegerOverflow=on
  Sum : Sum  Inputs=|+-
  Sum2 : Sum  Inputs=+++  SaturateOnIntegerOverflow=on  InputSameDT=on  OutDataTypeStr=Inherit: Same as first input
  Switch : Switch  Criteria=u2 > Threshold  Threshold=T_en
  To Workspace : ToWorkspace  Commented=on  VariableName=i_1  SampleTime=-1
  To Workspace1 : ToWorkspace  VariableName=i_dc1  SampleTime=-1
  To Workspace2 : ToWorkspace  VariableName=v_dc1  SampleTime=-1
  To Workspace3 : ToWorkspace  VariableName=i_dc_del1  SampleTime=-1
  Transfer Fcn1 : TransferFcn  Numerator=[w_f]  Denominator=[1 w_f]
  Transfer Fcn4 : TransferFcn  Numerator=[w_f]  Denominator=[1 w_f]
  Universal Bridge : powerlib/Power Electronics/Universal Bridge  Arms=3  SnubberResistance=1e5  SnubberCapacitance=inf  Device=Average-model based VSC  Ron=1e-3  Lon=0  ForwardVoltages="[  0  0  ]"  ForwardVoltage=0  GTOparameters=[ 10e-6 , 20e-6 ]  IGBTparameters=[ 1e-6 , 2e-6 ]  Measurements=None  Measurements_2=None  converterType=Rectifier
  Voltage Loop : Subsystem
  Voltage Measurement{,1..6} (7 alike) : powerlib/Measurements/Voltage Measurement  PhasorSimulation=off  OutputType=Complex  PSBequivalent=0
  abc to dq{1..6} (6 alike) : powerlib_meascontrol/Transformations/abc to dq0  Alignment=90 degrees behind phase A axis
  ac current limitation : Subsystem
  dq0 to abc : powerlib_meascontrol/Transformations/dq0 to abc  Alignment=90 degrees behind phase A axis
  d²2 : Product  SaturateOnIntegerOverflow=on  RndMeth=Zero  InputSameDT=on  OutDataTypeStr=Inherit: Same as first input
  i_dc1 : powerlib/Electrical Sources/Controlled Current Source  Initialize=off  Source_Type=DC  Amplitude=i_dc  Phase=0  Frequency=0  Measurements=None
  power set-point modification : Subsystem
  q²4 : Product  SaturateOnIntegerOverflow=on  RndMeth=Zero  InputSameDT=on  OutDataTypeStr=Inherit: Same as first input
  q²5 : Product  SaturateOnIntegerOverflow=on  RndMeth=Zero  InputSameDT=on  OutDataTypeStr=Inherit: Same as first input
  C : PMIOPort  Side=Right
  B : PMIOPort  Port=2  Side=Right
  A : PMIOPort  Port=3  Side=Right
  f : Outport
  V : Outport  Port=2
  P : Outport  Port=3
  Theta : Outport  Port=4
  wires:
  Rate Transition2/1 -> To Workspace2/1
  Switch/1 -> i_dc1/1, Rate Transition1/1
  Rate Transition1/1 -> To Workspace1/1
  Transfer Fcn1/1 -> Sum/2
  Constant3/1 -> power set-point modification/2(i_thr)
  Sum/1 -> [P_set]
  ac current limitation/3(||i_s_ref_dq0_lim||) -> Mux6/1
  Constant4/1 -> ac current limitation/2(i_max)
  ac current limitation/2(||i_s_ref_dq0||) -> Mux6/2
  Voltage Loop/1(i_s_ref_dq0) -> ac current limitation/1(i_s_ref_dq0)
  ac current limitation/1(i_s_ref_dq0_lim) -> Current Loop/1(i_s_ref_dq0)
  Gain2/1 -> Scope1/1
  Mux6/1 -> Gain2/1
  Add2/1 -> Transfer Fcn4/1
  Transfer Fcn4/1 -> Gain14/1
  [i_s_dq0] -> power set-point modification/1(i_s_dq0)
  power set-point modification/1(delta P*) -> Transfer Fcn1/1
  Gain1/1 -> Sum/1
  Pset/1 -> Gain1/1
  [v_dc] -> Gain17/1
  [P_s_abc] -> Add2/1
  Add6/1 -> Gain16/1
  [v_dc] -> Add6/2
  Gain17/1 -> Add4/3
  Constant1/1 -> Add6/1
  Gain16/1 -> Add4/1
  Gain13/1 -> Add4/2
  [P_set] -> Gain13/1
  Gain14/1 -> Add4/4
  [P_abc] -> Add2/2
  [P_set] -> Droop Control/3(p_set)
  Droop Control/1(w_ref) -> [w]
  Droop Control/2(theta_ref) -> [theta]
  [v_abc] -> Droop Control/5(V_abc)
  Constant9/1 -> Droop Control/4(v_m)
  [P_abc] -> Droop Control/2(p_m)
  Droop Control/3(v_ref_dq0) -> [v_ref_dq0]
  Constant11/1 -> Droop Control/1(w_b)
  [v_s_ref_dq0] -> dq0 to abc/1
  Gain19/1 -> Universal Bridge/1
  [v_dq0] -> Voltage Loop/2(v_dq0)
  [w] -> Voltage Loop/4(w)
  Current Loop/1(v_s_ref_dq0) -> [v_s_ref_dq0]
  [i_s_dq0] -> Current Loop/3(i_s_dq0)
  [v_dq0] -> Current Loop/2(v_dq0)
  [i_dq0] -> Voltage Loop/3(i_dq0)
  [v_ref_dq0] -> Voltage Loop/1(v_ref_dq0)
  [w] -> Current Loop/4(w)
  dq0 to abc/1 -> Gain19/1
  Memory1/1 -> [i_s_abc]
  Memory/1 -> [v_s_abc]
  Memory4/1 -> [v_dc], Rate Transition2/1
  Voltage Measurement/1 -> Memory4/1
  Memory3/1 -> [i_abc]
  Memory2/1 -> [v_abc]
  Mux4/1 -> Memory1/1
  Sqrt2/1 -> [V]
  Demux2/1 -> d²2/2, d²2/1  "d"
  Demux2/2 -> q²4/2, q²4/1  "q"
  d²2/1 -> Sum2/1
  Demux2/3 -> q²5/2, q²5/1  "0"
  Sum2/1 -> Sqrt2/1
  q²5/1 -> Sum2/3
  [v_dq0] -> Demux2/1
  q²4/1 -> Sum2/2
  [theta] -> dq0 to abc/2
  abc to dq6/1 -> [v_dq0]
  abc to dq5/1 -> [v_s_dq0]
  abc to dq4/1 -> [i_s_dq0]
  abc to dq3/1 -> [i_dq0]
  [theta] -> abc to dq3/2, abc to dq6/2, abc to dq5/2, abc to dq4/2
  [v_s_abc] -> abc to dq5/1
  [v_abc] -> abc to dq6/1
  [i_s_abc] -> abc to dq4/1
  [i_abc] -> abc to dq3/1
  [theta] -> Theta/1
  Gain4/1 -> V/1
  [i_abc] -> abc to dq1/1
  "Power (dq0, Instantaneous)"/1 -> [P_abc]
  "Power (dq0, Instantaneous)"/2 -> [Q_abc]
  [v_abc] -> abc to dq2/1
  [theta] -> abc to dq1/2, abc to dq2/2
  abc to dq2/1 -> "Power (dq0, Instantaneous)"/1
  abc to dq1/1 -> "Power (dq0, Instantaneous)"/2
  Mux1/1 -> Memory/1
  Mux3/1 -> Memory3/1
  Mux2/1 -> Memory2/1
  [w] -> Gain12/1
  Gain12/1 -> f/1
  [V] -> Gain4/1
  Voltage Measurement1/1 -> Mux1/1
  Voltage Measurement2/1 -> Mux1/2
  Voltage Measurement3/1 -> Mux1/3
  Voltage Measurement6/1 -> Mux2/3
  Voltage Measurement5/1 -> Mux2/2
  Voltage Measurement4/1 -> Mux2/1
  Current Measurement1/1 -> Mux3/1
  Current Measurement2/1 -> Mux3/2
  Current Measurement3/1 -> Mux3/3
  Current Measurement4/1 -> Mux4/1
  Current Measurement5/1 -> Mux4/2
  Current Measurement6/1 -> Mux4/3
  [P_abc] -> Gain7/1
  Gain7/1 -> P/1
  Saturation/1 -> Switch/1, Scope2/1
  Clock/1 -> Switch/2
  Add4/1 -> LTI System3/1
  From10/1 -> Demux1/1
  Demux1/1 -> Product1/2, Product1/1
  Product1/1 -> Minus4/1
  Demux1/3 -> Product7/1, Product7/2
  Minus4/1 -> Sqrt1/1
  Demux1/2 -> Product2/1, Product2/2
  Product7/1 -> Minus4/3
  Rate Transition/1 -> To Workspace/1
  Sqrt1/1 -> Rate Transition/1
  Product2/1 -> Minus4/2
  Rate Transition3/1 -> To Workspace3/1
  LTI System3/1 -> Saturation/1, Rate Transition3/1, Scope2/2, Switch/3
  connections:
  RL_c/RConn1 -- C_c1/LConn1 -- Current Measurement1/LConn1 -- Voltage Measurement4/LConn1
  C_c1/RConn1 -- Ground2/LConn1 -- C_a/RConn1 -- C_b/RConn1
  i_dc1/LConn1 -- G_dc1/RConn1 -- C_dc1/RConn1 -- Voltage Measurement/LConn2 -- Universal Bridge/RConn2
  Voltage Measurement1/LConn1 -- Current Measurement4/LConn1 -- Universal Bridge/LConn1
  Voltage Measurement2/LConn1 -- Current Measurement5/LConn1 -- Universal Bridge/LConn2
  Voltage Measurement3/LConn1 -- Universal Bridge/LConn3 -- Current Measurement6/LConn1
  Current Measurement1/RConn1 -- A/RConn1
  Current Measurement2/RConn1 -- B/RConn1
  Current Measurement3/RConn1 -- C/RConn1
  Voltage Measurement3/LConn2 -- Voltage Measurement1/LConn2 -- Voltage Measurement2/LConn2 -- Ground/LConn1
  Ground1/LConn1 -- Voltage Measurement4/LConn2 -- Voltage Measurement5/LConn2 -- Voltage Measurement6/LConn2
  i_dc1/RConn1 -- G_dc1/LConn1 -- C_dc1/LConn1 -- Universal Bridge/RConn1 -- Voltage Measurement/LConn1
  Current Measurement5/RConn1 -- RL_b/LConn1
  Current Measurement6/RConn1 -- RL_a/LConn1
  Current Measurement4/RConn1 -- RL_c/LConn1
  RL_a/RConn1 -- C_a/LConn1 -- Current Measurement3/LConn1 -- Voltage Measurement6/LConn1
  C_b/LConn1 -- Current Measurement2/LConn1 -- Voltage Measurement5/LConn1 -- RL_b/RConn1
